simulink model "mass_and_grad_est"  (R2022b)
settings: Solver=ode4  StartTime=0.0  StopTime=100  FixedStep=0.001  RelTol=1e-3
libraries: eeGeneralControl x1
settings Model: Creator=sriva  LastModifiedBy=sriva

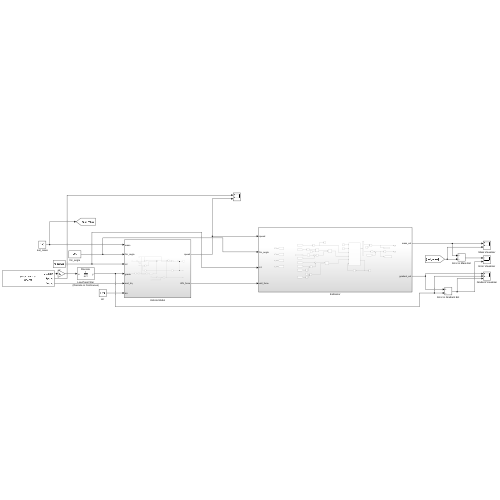
[thumbnail: Simulink's stored preview of the top-level diagram]
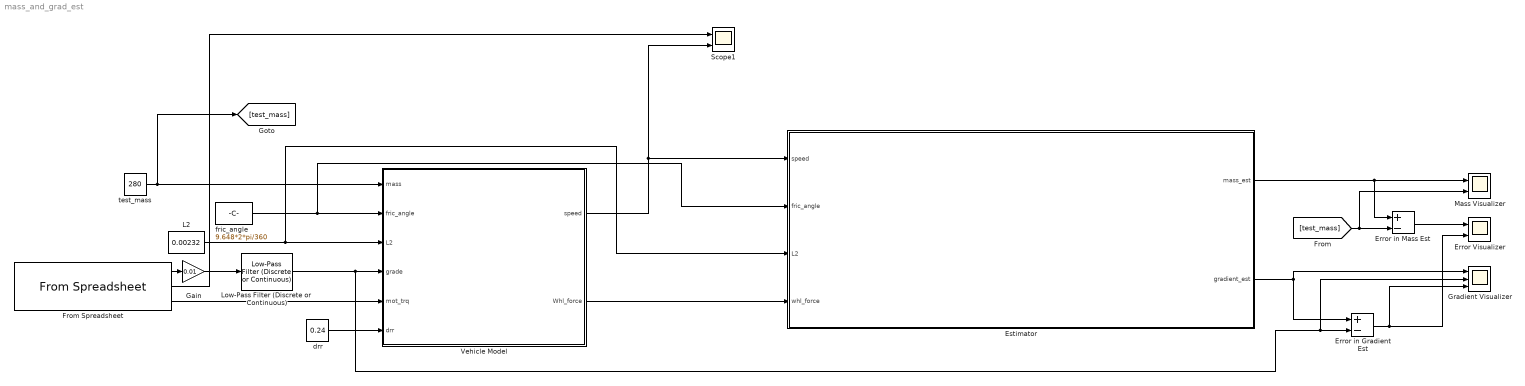
== system mass_and_grad_est ==
  Error Visualizer : Scope  NumInputPorts=2
  Error in Gradient Est : Sum  Inputs=+-
  Error in Mass Est : Sum  Inputs=+-
  Estimator : Subsystem
  From Spreadsheet : FromSpreadsheet  FileName=grade_def.xlsx
  Gain : Gain  Gain=0.01
  Gradient Visualizer : Scope  NumInputPorts=3
  L2 : Constant  Value=0.00232
  Low-Pass Filter (Discrete or Continuous) : eeGeneralControl/Low-Pass Filter (Discrete or Continuous)  K=1  T=1  B=inf  A=-inf  init_option=Inherited from block input  x0=0  Ts=-1
  Mass Visualizer : Scope  NumInputPorts=2
  Scope1 : Scope  NumInputPorts=2
  Vehicle Model : Subsystem
  drr : Constant  Value=0.24
  fric_angle : Constant  Value=9.648*2*pi/360
  test_mass : Constant  Value=280
  wires:
  fric_angle/1 -> Estimator/2(fric_angle), Vehicle Model/2(fric_angle)
  L2/1 -> Estimator/3(L2), Vehicle Model/3(L2)
  Vehicle Model/1(speed) -> Scope1/2, Estimator/1(speed)
  test_mass/1 -> [test_mass], Vehicle Model/1(mass)
  From Spreadsheet/3 -> Vehicle Model/5(mot_trq)
  drr/1 -> Vehicle Model/6(drr)
  From Spreadsheet/1 -> Gain/1
  Vehicle Model/2(Whl_force) -> Estimator/4(whl_force)
  Estimator/2(gradient_est) -> Error in Gradient Est/1, Gradient Visualizer/1
  From Spreadsheet/2 -> Scope1/1
  Estimator/1(mass_est) -> Error in Mass Est/1, Mass Visualizer/1
  Gain/1 -> Low-Pass Filter (Discrete or Continuous)/1
  Low-Pass Filter (Discrete or Continuous)/1 -> Error in Gradient Est/2, Gradient Visualizer/2, Vehicle Model/4(grade)
  Error in Gradient Est/1 -> Gradient Visualizer/3, Error Visualizer/2
  [test_mass] -> Mass Visualizer/2, Error in Mass Est/2
  Error in Mass Est/1 -> Error Visualizer/1

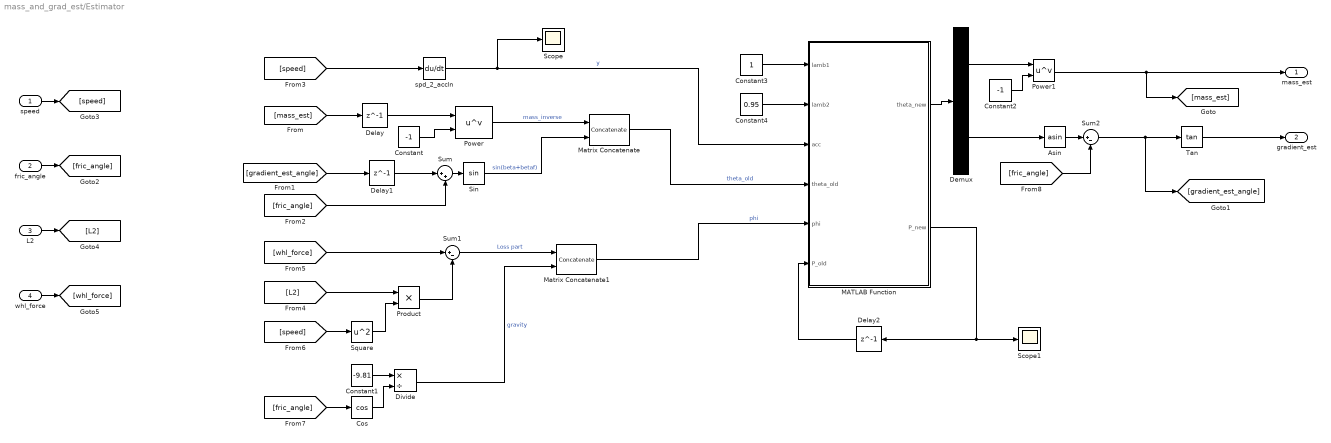
== system mass_and_grad_est/Estimator ==
  speed : Inport
  fric_angle : Inport  Port=2
  L2 : Inport  Port=3
  whl_force : Inport  Port=4
  Asin : Trigonometry  Operator=asin
  Constant : Constant  Value=-1
  Constant1 : Constant  Value=-9.81
  Constant2 : Constant  Value=-1
  Constant3 : Constant
  Constant4 : Constant  Value=0.95
  Cos : Trigonometry  Operator=cos
  Delay : Delay  DelayLength=1  InitialCondition=210
  Delay1 : Delay  DelayLength=1
  Delay2 : Delay  DelayLength=1  InitialCondition=[0.1,0;0,1]
  Demux : Demux  Outputs=2
  Divide : Product  Inputs=*/
  MATLAB Function : MATLAB Function  TreatAsAtomicUnit=on
  Matrix Concatenate : Concatenate  Mode=Multidimensional array  ConcatenateDimension=2
  Matrix Concatenate1 : Concatenate  Mode=Multidimensional array  ConcatenateDimension=2
  Power : Math  Operator=pow
  Power1 : Math  Operator=pow
  Product : Product
  Scope : Scope
  Scope1 : Scope
  Sin : Trigonometry
  Square : Math  Operator=square
  Sum : Sum  Inputs=|++
  Sum1 : Sum  Inputs=|+-
  Sum2 : Sum  Inputs=|+-
  Tan : Trigonometry  Operator=tan
  spd_2_accln : Derivative
  mass_est : Outport
  gradient_est : Outport  Port=2
  wires:
  Power1/1 -> [mass_est], mass_est/1
  Sum2/1 -> [gradient_est_angle], Tan/1
  [mass_est] -> Delay/1
  Delay/1 -> Power/1
  [gradient_est_angle] -> Delay1/1
  Delay1/1 -> Sum/1
  Constant/1 -> Power/2
  Power/1 -> Matrix Concatenate/1  "mass_inverse"
  fric_angle/1 -> [fric_angle]
  [fric_angle] -> Sum/2
  Sum/1 -> Sin/1
  Sin/1 -> Matrix Concatenate/2  "sin(beta+betaf)"
  Matrix Concatenate/1 -> MATLAB Function/4(theta_old)  "theta_old"
  speed/1 -> [speed]
  [speed] -> spd_2_accln/1
  L2/1 -> [L2]
  whl_force/1 -> [whl_force]
  [speed] -> Square/1
  [L2] -> Product/1
  Square/1 -> Product/2
  [whl_force] -> Sum1/1
  Product/1 -> Sum1/2
  Sum1/1 -> Matrix Concatenate1/1  "Loss part"
  [fric_angle] -> Cos/1
  Cos/1 -> Divide/2
  Constant1/1 -> Divide/1
  Divide/1 -> Matrix Concatenate1/2  "gravity"
  Matrix Concatenate1/1 -> MATLAB Function/5(phi)  "phi"
  spd_2_accln/1 -> Scope/1, MATLAB Function/3(acc)  "y"
  MATLAB Function/1(theta_new) -> Demux/1
  Demux/1 -> Power1/1
  Constant2/1 -> Power1/2
  Demux/2 -> Asin/1
  Asin/1 -> Sum2/1
  [fric_angle] -> Sum2/2
  MATLAB Function/2(P_new) -> Delay2/1, Scope1/1
  Delay2/1 -> MATLAB Function/6(P_old)
  Tan/1 -> gradient_est/1
  Constant3/1 -> MATLAB Function/1(lamb1)
  Constant4/1 -> MATLAB Function/2(lamb2)

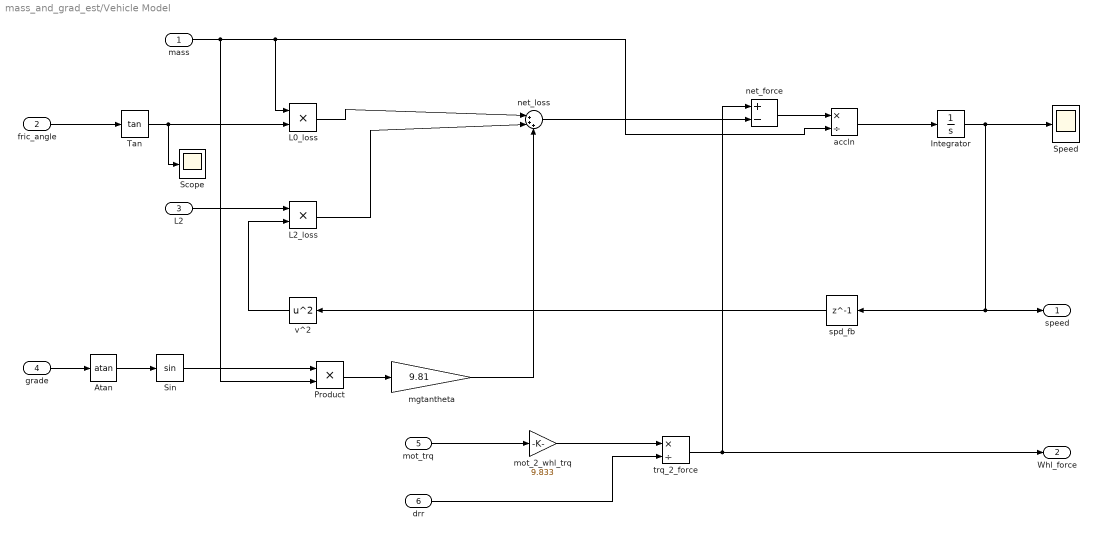
== system mass_and_grad_est/Vehicle Model ==
  mass : Inport
  fric_angle : Inport  Port=2
  L2 : Inport  Port=3
  grade : Inport  Port=4
  mot_trq : Inport  Port=5
  drr : Inport  Port=6
  Atan : Trigonometry  Operator=atan
  Integrator : Integrator
  L0_loss : Product
  L2_loss : Product
  Product : Product
  Scope : Scope
  Sin : Trigonometry
  Speed : Scope
  Tan : Trigonometry  Operator=tan
  accln : Product  Inputs=*/
  mgtantheta : Gain  Gain=9.81
  mot_2_whl_trq : Gain  Gain=9.833
  net_force : Sum  Inputs=+-
  net_loss : Sum  Inputs=|+++
  spd_fb : Delay  DelayLength=1  InitialCondition=0
  trq_2_force : Product  Inputs=*/
  v^2 : Math  Operator=square
  speed : Outport
  Whl_force : Outport  Port=2
  wires:
  mot_trq/1 -> mot_2_whl_trq/1
  mass/1 -> accln/2, L0_loss/1, Product/2
  L2/1 -> L2_loss/1
  L0_loss/1 -> net_loss/1
  L2_loss/1 -> net_loss/2
  mot_2_whl_trq/1 -> trq_2_force/1
  drr/1 -> trq_2_force/2
  trq_2_force/1 -> Whl_force/1, net_force/1
  net_loss/1 -> net_force/2
  v^2/1 -> L2_loss/2
  spd_fb/1 -> v^2/1
  net_force/1 -> accln/1
  accln/1 -> Integrator/1
  Integrator/1 -> Speed/1, speed/1, spd_fb/1
  grade/1 -> Atan/1
  Product/1 -> mgtantheta/1
  mgtantheta/1 -> net_loss/3
  fric_angle/1 -> Tan/1
  Tan/1 -> Scope/1, L0_loss/2
  Atan/1 -> Sin/1
  Sin/1 -> Product/1

== matlab function mass_and_grad_est/Estimator/MATLAB Function ==
  data: lamb1 input; lamb2 input; acc input; theta_new output; theta_old input; phi input; P_old input; P_new output
function [theta_new,P_new] = fcn(lamb1, lamb2, acc, theta_old, phi, P_old)

theta_old = theta_old';
phi = phi';
y = acc;
lamb = [lamb1, 0; 0, lamb2];

err = y - phi'*theta_old;
L_new = P_old*phi*((1+phi'*P_old*phi)^-1);

P_new = (lamb^-1)*([1,0;0,1]-L_new*phi')*P_old*(lamb^-1);

theta_new = theta_old+L_new*err;
